simulink model "firstSim"  (R2017b)
settings: Solver=VariableStepAuto  StartTime=0.0  StopTime=Tf  MaxStep=1e-2  RelTol=1e-3
values from neighbouring files (symbols this model uses):
  A = zeros(2,2,na,nV)    [linearization_toshare.m]    (also in missileLinearize.m = 0.196349540849)
  d = 0.5    [linearization_toshare.m]    (also in missileLinearize.m)
  Iyy = 49.4    [linearization_toshare.m]    (also in missileLinearize.m)
  m = 250    [linearization_toshare.m]    (also in missileLinearize.m)
  rho = 0.0023769    [linearization_toshare.m]    (also in missileLinearize.m)
  x0 = [0;0;3050]    [linearization_toshare.m]    (also in missileLinearize.m = x0bar+x0Pert)
settings Model: Creator=Andy  LastModifiedBy=pjseiler

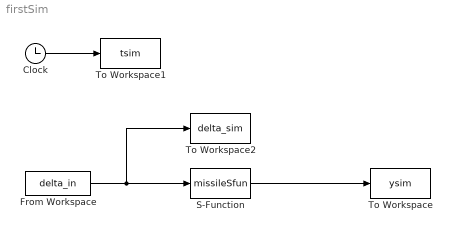
== system firstSim ==
  Clock : Clock
  From Workspace : FromWorkspace  VariableName=delta_in  SampleTime=0
  S-Function : S-Function  FunctionName=missileSfun  Parameters=x0,rho,d,A,m,Iyy  SFunctionDeploymentMode=off  EnableBusSupport=off
  To Workspace : ToWorkspace  VariableName=ysim  SampleTime=-1
  To Workspace1 : ToWorkspace  VariableName=tsim  SampleTime=-1
  To Workspace2 : ToWorkspace  VariableName=delta_sim  SampleTime=-1
  wires:
  S-Function/1 -> To Workspace/1
  From Workspace/1 -> To Workspace2/1, S-Function/1
  Clock/1 -> To Workspace1/1
